simulink model "step3"  (Simulink 10.2)
settings: Solver=ode113  StartTime=0.0  StopTime=5  RelTol=RT  AbsTol=AT  EnableMultiTasking=on
values from neighbouring files (symbols this model uses):
  F = [Fx;Fy;Mz]    [Jacobi_T.m]    (also in PRBDM_CTC_task.m = M_tilda*v+C_tilda*dX+G_tilda; RRR_CTC_task.m = M_tilda*v+V_tilda*dX+G_tilda; RRR_jtraj.m = q0; step2.mat = 10)
  gama0 = Rparams4dyn(3)    [PRBDM_3R_Dynamic_Matrices_Lagrange.m]    (also in PRBDM_3R_Dynamics.m = in4dyn(12); PRBDM_3R_Dynamics00.m = in4dyn(12); PRBDM_3R_DynamicsPID.m = in4dyn(12); PRBDM_3R_parameters.m = 0.1)
  gama1 = x(7)    [Jacobi_T.m]    (also in PRBDM_3R_Dynamic_Matrices_Lagrange.m = Rparams4dyn(4); PRBDM_3R_Dynamics.m = in4dyn(13); PRBDM_3R_Dynamics00.m = in4dyn(13); PRBDM_3R_DynamicsPID.m = in4dyn(13))
  gama2 = x(8)    [Jacobi_T.m]    (also in PRBDM_3R_Dynamic_Matrices_Lagrange.m = Rparams4dyn(5); PRBDM_3R_Dynamics.m = in4dyn(14); PRBDM_3R_Dynamics00.m = in4dyn(14); PRBDM_3R_DynamicsPID.m = in4dyn(14))
  gama3 = x(9)    [Jacobi_T.m]    (also in PRBDM_3R_Dynamic_Matrices_Lagrange.m = Rparams4dyn(6); PRBDM_3R_Dynamics.m = in4dyn(15); PRBDM_3R_Dynamics00.m = in4dyn(15); PRBDM_3R_DynamicsPID.m = in4dyn(15))
  k1 = Rparams4dyn(7)    [PRBDM_3R_Dynamic_Matrices_Lagrange.m]    (also in PRBDM_3R_Dynamics.m = in4dyn(16); PRBDM_3R_Dynamics00.m = in4dyn(16); PRBDM_3R_DynamicsPID.m = in4dyn(16); PRBDM_3R_parameters.m = 0.290628)
  k2 = Rparams4dyn(8)    [PRBDM_3R_Dynamic_Matrices_Lagrange.m]    (also in PRBDM_3R_Dynamics.m = in4dyn(17); PRBDM_3R_Dynamics00.m = in4dyn(17); PRBDM_3R_DynamicsPID.m = in4dyn(17); PRBDM_3R_parameters.m = 0.247572)
  k3 = Rparams4dyn(9)    [PRBDM_3R_Dynamic_Matrices_Lagrange.m]    (also in PRBDM_3R_Dynamics.m = in4dyn(18); PRBDM_3R_Dynamics00.m = in4dyn(18); PRBDM_3R_DynamicsPID.m = in4dyn(18); PRBDM_3R_parameters.m = 0.213624)
  L1 = z(8)    [Forward_kinematics.m]    (also in GeometricCalculation_simulink.m = Geoparams(5); Jacobi.m = x(4); PRBDM_3R_CTC.m = x(19); PRBDM_3R_Dynamic_Matrices_NewtonEular.m = robot_params(4))
  L2 = z(9)    [Forward_kinematics.m]    (also in GeometricCalculation_simulink.m = Geoparams(6); Jacobi.m = x(5); PRBDM_3R_CTC.m = x(20); PRBDM_3R_Dynamic_Matrices_NewtonEular.m = robot_params(5))
  L3 = z(10)    [Forward_kinematics.m]    (also in GeometricCalculation_simulink.m = Geoparams(7); Jacobi.m = x(6); PRBDM_3R_CTC.m = x(21); PRBDM_3R_Dynamic_Matrices_NewtonEular.m = robot_params(6))
  m1 = x(16)    [PRBDM_3R_CTC.m]    (also in PRBDM_3R_Dynamic_Matrices_NewtonEular.m = robot_params(1); PRBDM_3R_parameters.m = 0.35; PRBDM_3R_parameters.mat = 0.35; PRBDM_3R_test001.m = 0.1)
  m2 = x(17)    [PRBDM_3R_CTC.m]    (also in PRBDM_3R_Dynamic_Matrices_NewtonEular.m = robot_params(2); PRBDM_3R_parameters.m = 0.4; PRBDM_3R_parameters.mat = 0.4; PRBDM_3R_test001.m = 0.1)
  m3 = x(18)    [PRBDM_3R_CTC.m]    (also in PRBDM_3R_Dynamic_Matrices_NewtonEular.m = robot_params(3); PRBDM_3R_parameters.m = 0.15; PRBDM_3R_parameters.mat = 0.15; PRBDM_3R_test001.m = 0.1)
  Mz = x(6)    [Jacobi_T.m]    (also in step2.mat = 10; step2_trajectory.m = 10; step3.m = 10)
  W = x(22)    [PRBDM_3R_CTC.m]    (also in PRBDM_3R_Dynamic_Matrices_NewtonEular.m = robot_params(7); PRBDM_3R_Dynamics.m = in4dyn(20); PRBDM_3R_Dynamics00.m = in4dyn(20); PRBDM_3R_DynamicsPID.m = in4dyn(20))
settings Model: Creator=sayar  LastModifiedBy=Master
settings SolverCC: AutoScaleAbsTol=off
settings DataIOCC: SignalLoggingSaveFormat=Dataset  Refine=RF
settings OptimizationCC: ExpressionDepthLimit=2147483647
settings DebuggingCC: SolverPrmCheckMsg=warning  StateNameClashWarn=warning

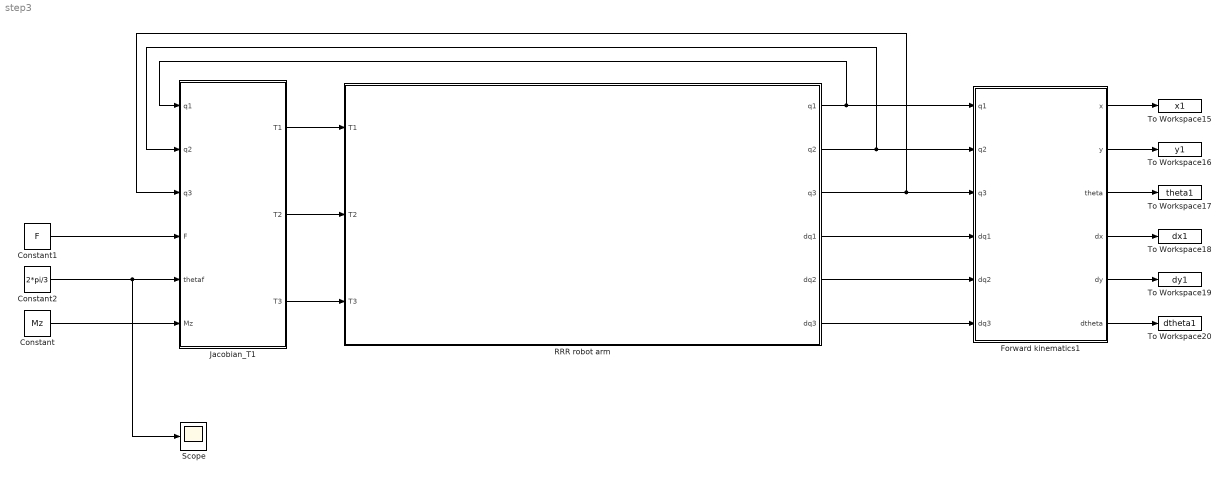
== system step3 ==
  Constant : Constant  Value=Mz
  Constant1 : Constant  Value=F
  Constant2 : Constant  Value=2*pi/3
  Forward kinematics1 : Subsystem
  Jacobian_T1 : Subsystem
  RRR robot arm : Subsystem
      mask Display: image(imread('RRR.png'))
  Scope : Scope
  To Workspace15 : ToWorkspace  VariableName=x1  SampleTime=-1
  To Workspace16 : ToWorkspace  VariableName=y1  SampleTime=-1
  To Workspace17 : ToWorkspace  VariableName=theta1  SampleTime=-1
  To Workspace18 : ToWorkspace  VariableName=dx1  SampleTime=-1
  To Workspace19 : ToWorkspace  VariableName=dy1  SampleTime=-1
  To Workspace20 : ToWorkspace  VariableName=dtheta1  SampleTime=-1
  wires:
  Forward kinematics1/6(dtheta) -> To Workspace20/1
  Forward kinematics1/1(x) -> To Workspace15/1
  Forward kinematics1/3(theta) -> To Workspace17/1
  RRR robot arm/1(q1) -> Forward kinematics1/1(q1), Jacobian_T1/1(q1)
  RRR robot arm/5(dq2) -> Forward kinematics1/5(dq2)
  Jacobian_T1/3(T3) -> RRR robot arm/3(T3)
  RRR robot arm/6(dq3) -> Forward kinematics1/6(dq3)
  Forward kinematics1/4(dx) -> To Workspace18/1
  Forward kinematics1/2(y) -> To Workspace16/1
  Forward kinematics1/5(dy) -> To Workspace19/1
  Jacobian_T1/2(T2) -> RRR robot arm/2(T2)
  RRR robot arm/4(dq1) -> Forward kinematics1/4(dq1)
  Jacobian_T1/1(T1) -> RRR robot arm/1(T1)
  RRR robot arm/3(q3) -> Forward kinematics1/3(q3), Jacobian_T1/3(q3)
  RRR robot arm/2(q2) -> Forward kinematics1/2(q2), Jacobian_T1/2(q2)
  Constant2/1 -> Scope/1, Jacobian_T1/5(thetaf)
  Constant/1 -> Jacobian_T1/6(Mz)
  Constant1/1 -> Jacobian_T1/4(F)

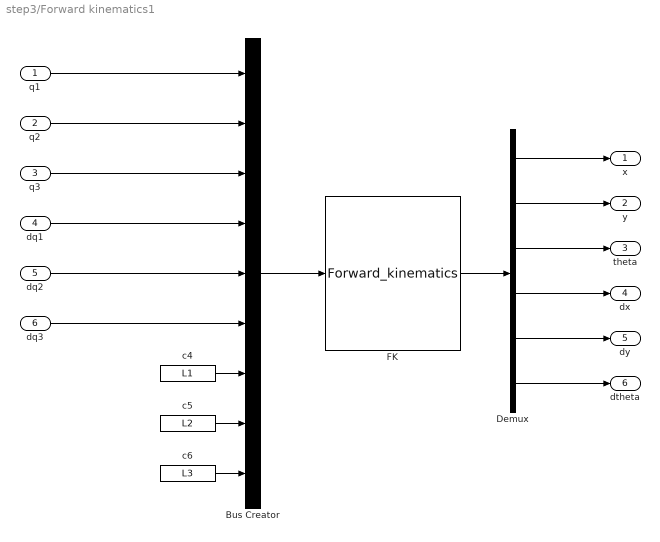
== system step3/Forward kinematics1 ==
  q1 : Inport
  q2 : Inport  Port=2
  q3 : Inport  Port=3
  dq1 : Inport  Port=4
  dq2 : Inport  Port=5
  dq3 : Inport  Port=6
  Bus Creator : BusCreator  Inputs=9
  Demux : Demux  Outputs=6
  FK : MATLABFcn  MATLABFcn=Forward_kinematics  OutputDimensions=6
  c4 : Constant  Value=L1
  c5 : Constant  Value=L2
  c6 : Constant  Value=L3
  x : Outport
  y : Outport  Port=2
  theta : Outport  Port=3
  dx : Outport  Port=4
  dy : Outport  Port=5
  dtheta : Outport  Port=6
  wires:
  c6/1 -> Bus Creator/9
  Demux/1 -> x/1
  Demux/4 -> dx/1
  c4/1 -> Bus Creator/7
  Demux/5 -> dy/1
  q2/1 -> Bus Creator/2
  q1/1 -> Bus Creator/1
  q3/1 -> Bus Creator/3
  Bus Creator/1 -> FK/1
  dq2/1 -> Bus Creator/5
  Demux/2 -> y/1
  FK/1 -> Demux/1
  dq1/1 -> Bus Creator/4
  Demux/3 -> theta/1
  dq3/1 -> Bus Creator/6
  Demux/6 -> dtheta/1
  c5/1 -> Bus Creator/8

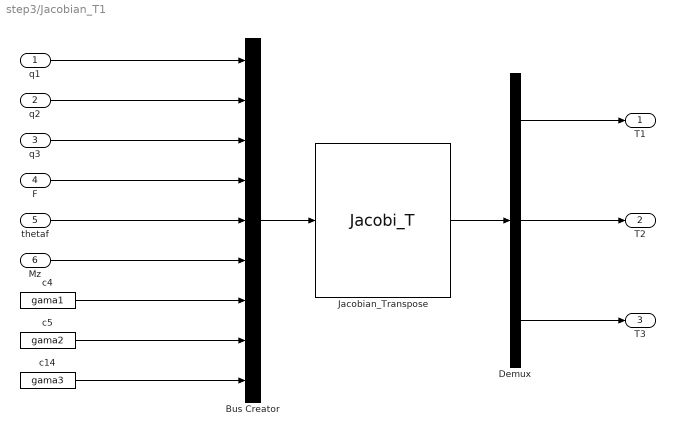
== system step3/Jacobian_T1 ==
  q1 : Inport
  q2 : Inport  Port=2
  q3 : Inport  Port=3
  F : Inport  Port=4
  thetaf : Inport  Port=5
  Mz : Inport  Port=6
  Bus Creator : BusCreator  Inputs=9
  Demux : Demux  Outputs=3
  Jacobian_Transpose : MATLABFcn  MATLABFcn=Jacobi_T  OutputDimensions=3
  c14 : Constant  Value=gama3
  c4 : Constant  Value=gama1
  c5 : Constant  Value=gama2
  T1 : Outport
  T2 : Outport  Port=2
  T3 : Outport  Port=3
  wires:
  Jacobian_Transpose/1 -> Demux/1
  Demux/2 -> T2/1
  Bus Creator/1 -> Jacobian_Transpose/1
  Demux/1 -> T1/1
  Demux/3 -> T3/1
  F/1 -> Bus Creator/4
  thetaf/1 -> Bus Creator/5
  Mz/1 -> Bus Creator/6
  q1/1 -> Bus Creator/1
  q2/1 -> Bus Creator/2
  q3/1 -> Bus Creator/3
  c5/1 -> Bus Creator/8
  c14/1 -> Bus Creator/9
  c4/1 -> Bus Creator/7

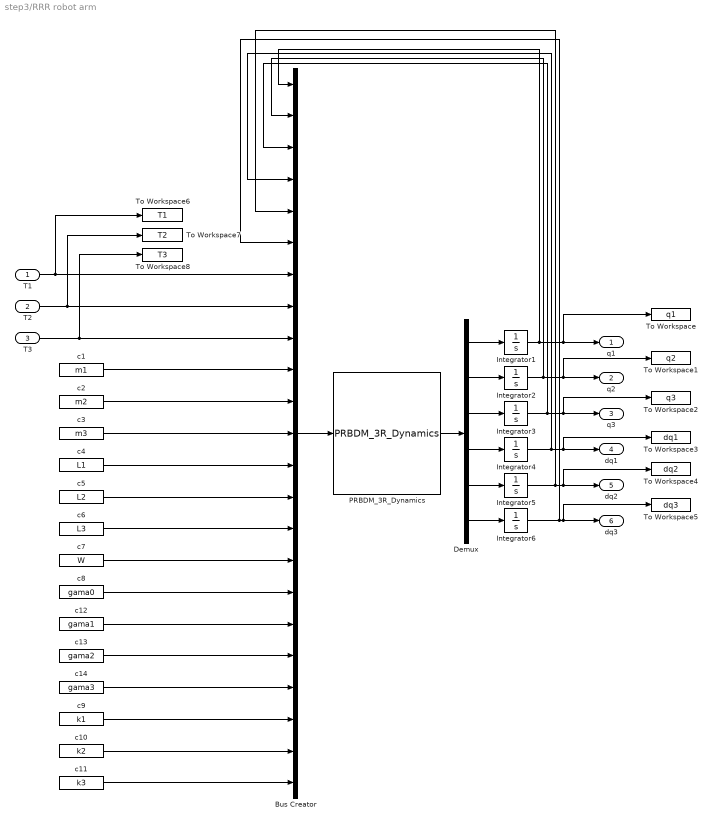
== system step3/RRR robot arm ==
  T1 : Inport
  T2 : Inport  Port=2
  T3 : Inport  Port=3
  Bus Creator : BusCreator  Inputs=23
  Demux : Demux  Outputs=6
  Integrator{1,4..6} (4 alike) : Integrator
  Integrator2 : Integrator  InitialCondition=3*pi/4
  Integrator3 : Integrator  InitialCondition=-3*pi/4
  PRBDM_3R_Dynamics : MATLABFcn  MATLABFcn=PRBDM_3R_Dynamics  OutputDimensions=6
  To Workspace : ToWorkspace  VariableName=q1  SampleTime=-1
  To Workspace1 : ToWorkspace  VariableName=q2  SampleTime=-1
  To Workspace2 : ToWorkspace  VariableName=q3  SampleTime=-1
  To Workspace3 : ToWorkspace  VariableName=dq1  SampleTime=-1
  To Workspace4 : ToWorkspace  VariableName=dq2  SampleTime=-1
  To Workspace5 : ToWorkspace  VariableName=dq3  SampleTime=-1
  To Workspace6 : ToWorkspace  VariableName=T1  SampleTime=-1
  To Workspace7 : ToWorkspace  VariableName=T2  SampleTime=-1
  To Workspace8 : ToWorkspace  VariableName=T3  SampleTime=-1
  c1 : Constant  Value=m1
  c10 : Constant  Value=k2
  c11 : Constant  Value=k3
  c12 : Constant  Value=gama1
  c13 : Constant  Value=gama2
  c14 : Constant  Value=gama3
  c2 : Constant  Value=m2
  c3 : Constant  Value=m3
  c4 : Constant  Value=L1
  c5 : Constant  Value=L2
  c6 : Constant  Value=L3
  c7 : Constant  Value=W
  c8 : Constant  Value=gama0
  c9 : Constant  Value=k1
  q1 : Outport
  q2 : Outport  Port=2
  q3 : Outport  Port=3
  dq1 : Outport  Port=4
  dq2 : Outport  Port=5
  dq3 : Outport  Port=6
  wires:
  Demux/1 -> Integrator1/1
  Demux/2 -> Integrator2/1
  Demux/3 -> Integrator3/1
  Demux/4 -> Integrator4/1
  Demux/5 -> Integrator5/1
  Demux/6 -> Integrator6/1
  Integrator1/1 -> Bus Creator/1, q1/1, To Workspace/1
  Integrator2/1 -> Bus Creator/2, q2/1, To Workspace1/1
  Integrator3/1 -> Bus Creator/3, q3/1, To Workspace2/1
  Integrator4/1 -> Bus Creator/4, dq1/1, To Workspace3/1
  Integrator5/1 -> Bus Creator/5, dq2/1, To Workspace4/1
  Integrator6/1 -> Bus Creator/6, dq3/1, To Workspace5/1
  c1/1 -> Bus Creator/10
  c2/1 -> Bus Creator/11
  PRBDM_3R_Dynamics/1 -> Demux/1
  Bus Creator/1 -> PRBDM_3R_Dynamics/1
  T3/1 -> To Workspace8/1, Bus Creator/9
  T2/1 -> To Workspace7/1, Bus Creator/8
  T1/1 -> To Workspace6/1, Bus Creator/7
  c3/1 -> Bus Creator/12
  c4/1 -> Bus Creator/13
  c5/1 -> Bus Creator/14
  c6/1 -> Bus Creator/15
  c7/1 -> Bus Creator/16
  c8/1 -> Bus Creator/17
  c12/1 -> Bus Creator/18
  c13/1 -> Bus Creator/19
  c14/1 -> Bus Creator/20
  c9/1 -> Bus Creator/21
  c10/1 -> Bus Creator/22
  c11/1 -> Bus Creator/23
